simulink subsystem "euler_eqn"  (R2022b)
settings: Solver=VariableStepAuto  StartTime=0.0  StopTime=10.0  RelTol=1e-3
undefined symbols (not defined in the file or in its folder): gainx, gainy, gainz, Ix, Iy, Iz, w0
settings Model: Creator=brent  LastModifiedBy=brent

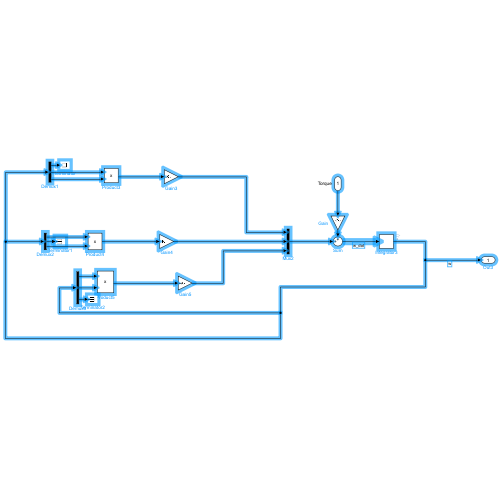
[thumbnail: Simulink's stored preview of the top-level diagram]
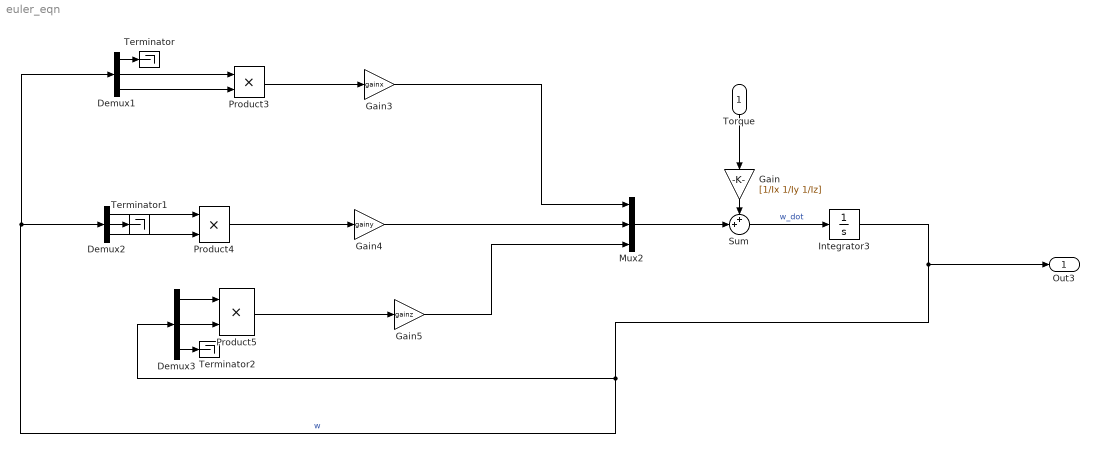
== system euler_eqn ==
  Torque : Inport
  Demux1 : Demux  Outputs=3
  Demux2 : Demux  Outputs=3
  Demux3 : Demux  Outputs=3
  Gain : Gain  Gain=[1/Ix 1/Iy 1/Iz]
  Gain3 : Gain  Gain=gainx
  Gain4 : Gain  Gain=gainy
  Gain5 : Gain  Gain=gainz
  Integrator3 : Integrator  InitialCondition=w0
  Mux2 : Mux  Inputs=3
  Product3 : Product
  Product4 : Product
  Product5 : Product
  Sum : Sum  Inputs=++|
  Terminator : Terminator
  Terminator1 : Terminator
  Terminator2 : Terminator
  Out3 : Outport
  wires:
  Torque/1 -> Gain/1
  Demux2/2 -> Terminator1/1
  Demux3/3 -> Terminator2/1
  Demux1/3 -> Product3/2
  Demux2/1 -> Product4/1
  Gain/1 -> Sum/1
  Gain4/1 -> Mux2/2
  Demux1/2 -> Product3/1
  Gain5/1 -> Mux2/3
  Product4/1 -> Gain4/1
  Demux2/3 -> Product4/2
  Demux3/2 -> Product5/2
  Product5/1 -> Gain5/1
  Gain3/1 -> Mux2/1
  Integrator3/1 -> Out3/1, Demux1/1, Demux2/1, Demux3/1  "w"
  Product3/1 -> Gain3/1
  Demux1/1 -> Terminator/1
  Mux2/1 -> Sum/2
  Demux3/1 -> Product5/1
  Sum/1 -> Integrator3/1  "w_dot"
